simulink model "prblm7"  (R2020b)
settings: Solver=VariableStepAuto  StartTime=0.0  StopTime=10.0  RelTol=1e-3
settings Model: Creator=shridhar  LastModifiedBy=shridhar

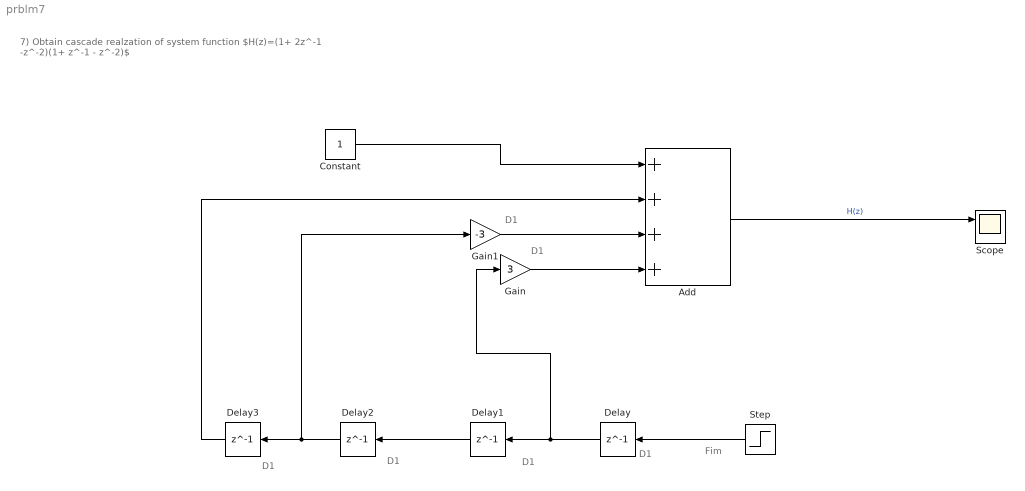
== system prblm7 ==
  note: D1
  note: D1
  note: D1
  note: D1
  note: D1
  note: D1
  note: Fim
  note: 7) Obtain cascade realzation of system function
      | $H(z)=(1+ 2z^-1 -z^-2)(1+ z^-1 - z^-2)$
  Add : Sum  Inputs=++++
  Constant : Constant
  Delay{,1..3} (4 alike) : Delay  DelayLength=1
  Gain : Gain  Gain=3
  Gain1 : Gain  Gain=-3
  Scope : Scope  NumInputPorts=2
  Step : Step  SampleTime=0
  wires:
  Add/1 -> Scope/1  "H(z)"
  Delay2/1 -> Gain1/1, Delay3/1
  Delay1/1 -> Delay2/1
  Delay/1 -> Gain/1, Delay1/1
  Step/1 -> Delay/1
  Gain/1 -> Add/4
  Gain1/1 -> Add/3
  Constant/1 -> Add/1
  Delay3/1 -> Add/2
